simulink model "chap4_10sim"  (Simulink 8.1)
settings: Solver=ode45  StartTime=0.0  StopTime=5  FixedStep=0.001  RelTol=1e-3
settings Model: Creator=ljk  LastModifiedBy=liujk  ExtModeTrigMode=oneshot  ExtModeArmWhenConnect=off
settings DataIOCC: LimitDataPoints=off  SignalLoggingName=sigsOut
settings OptimizationCC: BooleanDataType=off
settings DebuggingCC: SaveWithParameterizedLinksMsg=none  SignalResolutionControl=TryResolveAllWithWarning  SolverPrmCheckMsg=none  MultiTaskDSMMsg=warning  MultiTaskCondExecSysMsg=none  StrictBusMsg=None
settings HardwareCC: TargetUnknown=on
settings RTWCC: IncludeERTFirstTime=on

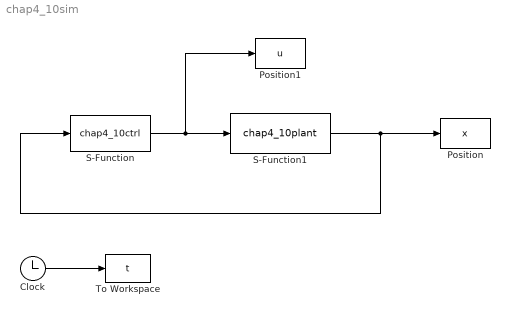
== system chap4_10sim ==
  Clock : Clock
  Position : ToWorkspace  VariableName=x  SampleTime=-1
  Position1 : ToWorkspace  VariableName=u  SampleTime=-1
  S-Function : S-Function  FunctionName=chap4_10ctrl  EnableBusSupport=off
  S-Function1 : S-Function  FunctionName=chap4_10plant  EnableBusSupport=off
  To Workspace : ToWorkspace  VariableName=t  SampleTime=-1
  wires:
  S-Function/1 -> S-Function1/1, Position1/1
  S-Function1/1 -> S-Function/1, Position/1
  Clock/1 -> To Workspace/1
